simulink model "DeMux1"  (R2024b)
settings: Solver=VariableStepAuto  StartTime=0.0  StopTime=10.0  RelTol=1e-3
settings Model: Creator=Ahmad  LastModifiedBy=Ahmad

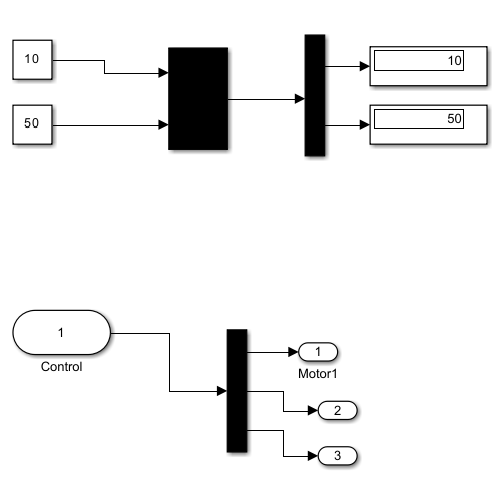
[thumbnail: Simulink's stored preview of the top-level diagram]
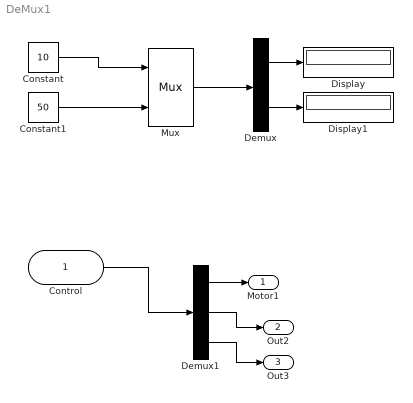
== system DeMux1 ==
  Control : Inport
  Constant : Constant  Value=10
  Constant1 : Constant  Value=50
  Demux : Demux  Outputs=2
  Demux1 : Demux  Outputs=3
  Display : Display
  Display1 : Display
  Mux : Mux  Inputs=2
  Motor1 : Outport
  Out2 : Outport  Port=2
  Out3 : Outport  Port=3
  wires:
  Mux/1 -> Demux/1
  Constant1/1 -> Mux/2
  Constant/1 -> Mux/1
  Demux/1 -> Display/1
  Demux/2 -> Display1/1
  Control/1 -> Demux1/1
  Demux1/1 -> Motor1/1
  Demux1/2 -> Out2/1
  Demux1/3 -> Out3/1
